simulink model "Sinpwmlithuyet"  (R2022b)
settings: Solver=VariableStepAuto  StartTime=0.0  StopTime=0.1  RelTol=1e-3
libraries: spsIGBTDiodeLib x6, simulink x3, spsThreePhaseSeriesRLCBranchLib x2, spsAsynchronousMachineSIUnitsLib x1, spsDCVoltageSourceLib x1, spsGroundLib x1, spsThreePhaseVIMeasurementLib x1, spsTriangleGeneratorLib x1, spspowerguiLib x1
settings Model: Creator=doand  LastModifiedBy=doand

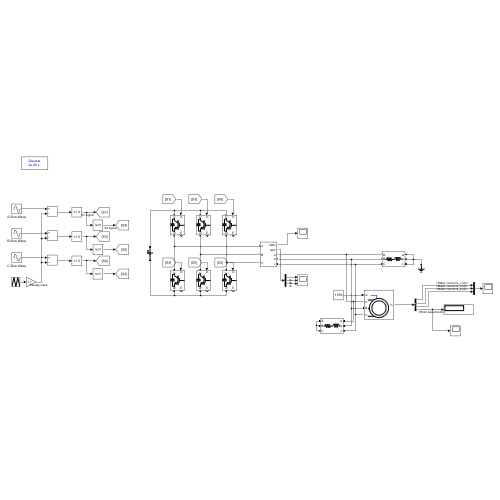
[thumbnail: Simulink's stored preview of the top-level diagram]
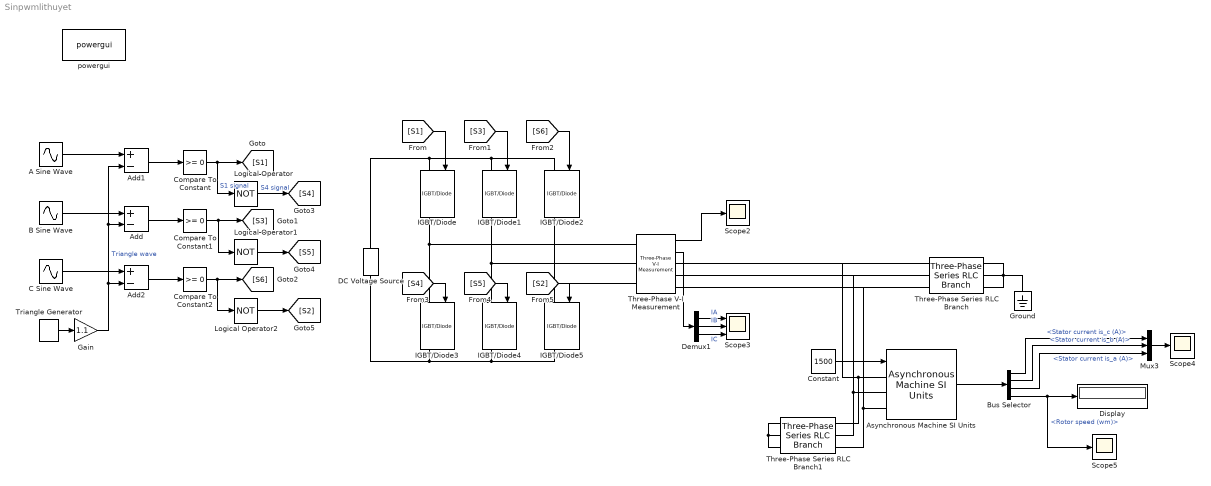
== system Sinpwmlithuyet ==
  A Sine Wave : Sin  Frequency=2*pi*50  SampleTime=0
  Add : Sum  Inputs=+-
  Add1 : Sum  Inputs=+-
  Add2 : Sum  Inputs=+-
  Asynchronous Machine SI Units : spsAsynchronousMachineSIUnitsLib/Asynchronous Machine SI Units  RotorType=Squirrel-cage  PresetModel=No  MechanicalLoad=Speed w  ShowDetailedParameters=on  ReferenceFrame=Rotor  Units=SI  MeasurementBus=off  NominalParameters=[1.845e+04 400 50]  VoltageRatio=1  Stator=[0.5968 0.0003495]  Rotor=[0.6258 0.005473]  Cage1=[0.4155 0.002066]  Cage2=[0.4168 0.0003495]  Lm=0.0354  Mechanical=[0.05 0.005879 2]  PolePairs=2  InitialConditions=[0 0 0 0 0 0 0 0]  SimulateSaturation=off  Saturation=[14.03593122, 27.81365428, 53.79336849, 72.68890987, 97.98006896, 148.6815601, 215.7428561, 302.9841135, 428.7778367 ; 230, 322, 414, 460, 506, 552, 598, 644, 690]  LoadFlowParameters=1492000  TsPowergui=0  TsBlock=-1  IterativeModel=Trapezoidal non iterative  IterativeDiscreteModel=Trapezoidal non iterative  Pmec=1.492e+006
  B Sine Wave : Sin  Frequency=2*pi*50  Phase=2*pi/3  SampleTime=0
  Bus Selector : BusSelector  OutputSignals=Stator measurements.Stator current is_c (A),Stator measurements.Stator current is_b (A),Stator measurements.Stator current is_a (A),Mechanical.Rotor speed (wm)
  C Sine Wave : Sin  Frequency=2*pi*50  Phase=-2*pi/3  SampleTime=0
  Compare To Constant : simulink/Logic and Bit Operations/Compare To Constant  relop=>=  const=0  OutDataTypeStr=boolean
  Compare To Constant1 : simulink/Logic and Bit Operations/Compare To Constant  relop=>=  const=0  OutDataTypeStr=boolean
  Compare To Constant2 : simulink/Logic and Bit Operations/Compare To Constant  relop=>=  const=0  OutDataTypeStr=boolean
  Constant : Constant  Value=1500
  DC Voltage Source : spsDCVoltageSourceLib/DC Voltage Source  Amplitude=270  Measurements=None
  Demux1 : Demux  Outputs=3
  Display : Display
  Gain : Gain  Gain=1.1
  Ground : spsGroundLib/Ground  LConnTagsString=a
  IGBT/Diode{,1..5} (6 alike) : spsIGBTDiodeLib/IGBT//Diode  Ron=1e-3  Rs=1e5  Cs=inf  Measurements=on
  Logical Operator : Logic  Operator=NOT  AllPortsSameDT=off  OutDataTypeStr=boolean
  Logical Operator1 : Logic  Operator=NOT  AllPortsSameDT=off  OutDataTypeStr=boolean
  Logical Operator2 : Logic  Operator=NOT  AllPortsSameDT=off  OutDataTypeStr=boolean
  Mux3 : Mux  Inputs=3
  Scope2 : Scope
  Scope3 : Scope  NumInputPorts=3
  Scope4 : Scope
  Scope5 : Scope
  Three-Phase Series RLC Branch : spsThreePhaseSeriesRLCBranchLib/Three-Phase Series RLC Branch  LConnTagsString=A|B|C  RConnTagsString=A|B|C  BranchType=RL  Resistance=1  Inductance=0.5  Capacitance=1e-6  Measurements=None
  Three-Phase Series RLC Branch1 : spsThreePhaseSeriesRLCBranchLib/Three-Phase Series RLC Branch  LConnTagsString=A|B|C  RConnTagsString=A|B|C  BranchType=RL  Resistance=500  Inductance=10  Capacitance=1e-6  Measurements=None
  Three-Phase V-I Measurement : spsThreePhaseVIMeasurementLib/Three-Phase V-I Measurement  VoltageMeasurement=phase-to-ground  SetLabelV=off  LabelV=Vabc  Vpu=off  VpuLL=off  CurrentMeasurement=yes  SetLabelI=off  LabelI=Iabc  Ipu=off  Pbase=100e6  Vbase=500e3  OutputType=Complex  PhasorSimulation=off  PSBequivalent=0
  Triangle Generator : spsTriangleGeneratorLib/Triangle Generator  Freq=2000*4  Phase=0  Ts=0
  powergui : spspowerguiLib/powergui  Priority=1  SimulationMode=Discrete  SampleTime=2e-8  frequency=50  Iterations=50  frequencyindice=0  Pbase=100e6  ErrMax=1e-4  UnitsV=kV  UnitsW=MW  buscounter=0  FunctionMessages=off  echomessages=off  EnableUseOfTLC=off  CurrentSourceSwitches=off  DisableSnubberDevices=off  DisableRonSwitches=off  DisableVfSwitches=off  DisplayEquations=off  AutomaticDiscreteSolvers=off  SolverType=Tustin/Backward Euler (TBE)  Interpol=off  ExternalGateDelay=off  methode=off  Ts=100  x0status=blocks  SPID=on  SwTol=0  HookPort=off  NonlinearTolerance=1e-4  nMaxIteration=100  ContinueOnMaxIteration=off  RestoreLinks=warning  ResistiveCurrentMeasurement=off  Frange=[0:2:500]  Ylog=off  Xlog=on  ShowGrid=off  save=off  variable=ZData  structure=0  ZoomFFT=off  StartTime=0.0  cycles=1  DisplayStyle=1  fundamental=60  FreqAxis=off  MaxFrequency=1000  frequencyindicesteady=1  RmsSteady=1  display=off
  wires:
  B Sine Wave/1 -> Add/1
  C Sine Wave/1 -> Add2/1
  A Sine Wave/1 -> Add1/1
  Gain/1 -> Add2/2, Add/2, Add1/2  "Triangle wave"
  Add1/1 -> Compare To Constant/1
  Add/1 -> Compare To Constant1/1
  Add2/1 -> Compare To Constant2/1
  Compare To Constant/1 -> Logical Operator/1, [S1]  "S1 signal"
  Compare To Constant1/1 -> Logical Operator1/1, [S3]
  Compare To Constant2/1 -> Logical Operator2/1, [S6]
  [S1] -> IGBT/Diode/1
  [S3] -> IGBT/Diode1/1
  [S6] -> IGBT/Diode2/1
  Logical Operator/1 -> [S4]  "S4 signal"
  Logical Operator1/1 -> [S5]
  Logical Operator2/1 -> [S2]
  [S4] -> IGBT/Diode3/1
  [S2] -> IGBT/Diode5/1
  [S5] -> IGBT/Diode4/1
  Three-Phase V-I Measurement/1 -> Scope2/1
  Three-Phase V-I Measurement/2 -> Demux1/1
  Demux1/3 -> Scope3/3  "IC"
  Demux1/2 -> Scope3/2  "IB"
  Triangle Generator/1 -> Gain/1
  Asynchronous Machine SI Units/1 -> Bus Selector/1
  Bus Selector/1 -> Mux3/1  "<Stator current is_c (A)>"
  Bus Selector/2 -> Mux3/2  "<Stator current is_b (A)>"
  Bus Selector/3 -> Mux3/3  "<Stator current is_a (A)>"
  Bus Selector/4 -> Scope5/1, Display/1  "<Rotor speed (wm)>"
  Constant/1 -> Asynchronous Machine SI Units/1
  Demux1/1 -> Scope3/1  "IA"
  Mux3/1 -> Scope4/1
  connections:
  DC Voltage Source/RConn1 -- IGBT/Diode/LConn1 -- IGBT/Diode2/LConn1 -- IGBT/Diode1/LConn1
  DC Voltage Source/LConn1 -- IGBT/Diode3/RConn1 -- IGBT/Diode5/RConn1 -- IGBT/Diode4/RConn1
  Three-Phase V-I Measurement/LConn1 -- IGBT/Diode/RConn1 -- IGBT/Diode3/LConn1
  Three-Phase V-I Measurement/LConn2 -- IGBT/Diode1/RConn1 -- IGBT/Diode4/LConn1
  Three-Phase V-I Measurement/LConn3 -- IGBT/Diode5/LConn1 -- IGBT/Diode2/RConn1
  Ground/LConn1 -- Three-Phase Series RLC Branch/RConn1 -- Three-Phase Series RLC Branch/RConn2 -- Three-Phase Series RLC Branch/RConn3
  Three-Phase Series RLC Branch1/RConn1 -- Three-Phase V-I Measurement/RConn1 -- Three-Phase Series RLC Branch/LConn1 -- Asynchronous Machine SI Units/LConn1
  Three-Phase Series RLC Branch1/RConn2 -- Three-Phase V-I Measurement/RConn2 -- Three-Phase Series RLC Branch/LConn2 -- Asynchronous Machine SI Units/LConn2
  Asynchronous Machine SI Units/LConn3 -- Three-Phase V-I Measurement/RConn3 -- Three-Phase Series RLC Branch/LConn3 -- Three-Phase Series RLC Branch1/RConn3
  Three-Phase Series RLC Branch1/LConn1 -- Three-Phase Series RLC Branch1/LConn3 -- Three-Phase Series RLC Branch1/LConn2
